simulink model "LKAS_Project"  (R2024b)
settings: Solver=ode45  StartTime=0.0  StopTime=T_final  RelTol=1e-3  EnableMultiTasking=on
undefined symbols (not defined in the file or in its folder): Calpha, Cf, Cr, driving, Izz, Kalpha, Ke, l, lf, lr, m, max_steer, mu, Tc, Vy0, X0, Y0, Yaw0, yaw_rate0
libraries: drivingscenarioandsensors x2
settings Model: Creator=user  LastModifiedBy=justi
settings SolverCC: ZeroCrossAlgorithm=Non-adaptive  AlgebraicLoopSolver=TrustRegion
settings DataIOCC: LimitDataPoints=on  SaveFormat=Array  SignalLoggingSaveFormat=ModelDataLogs  ReturnWorkspaceOutputs=off
settings OptimizationCC: ExpressionDepthLimit=2147483647  InitFltsAndDblsToZero=on  LifeSpan=inf
settings DebuggingCC: UnderspecifiedInitializationDetection=Classic  MergeDetectMultiDrivingBlocksExec=none  SolverPrmCheckMsg=warning  FcnCallInpInsideContextMsg=warning  UnconnectedInputMsg=warning  UnconnectedOutputMsg=warning  UnconnectedLineMsg=warning  StateNameClashWarn=warning  SFUnexpectedBacktrackingDiag=warning  SFNoUnconditionalDefaultTransitionDiag=warning  SFExecutionAtInitializationDiag=none  ArithmeticOperatorsInVariantConditions=warning
settings HardwareCC: ProdBitPerPointer=32  ProdBitPerSizeT=32  ProdBitPerPtrDiffT=32  ProdLargestAtomicFloat=None  ProdIntDivRoundTo=Undefined  ProdEndianess=Unspecified  ProdWordSize=32  ProdHWDeviceType=32-bit Generic
settings ModelReferenceCC: PropagateSignalLabelsOutOfModel=off
settings RTWCC: GPUComputeCapability=3.5
settings CodeAppCC: StateflowObjectComments=on
settings GRTTargetCC: TargetLangStandard=C89/C90 (ANSI)  CombineOutputUpdateFcns=off  GRTInterface=on
settings ConfigComp: CovMetricSettings=dw  CovSaveCumulativeToWorkspaceVar=on  CovSaveSingleToWorkspaceVar=on

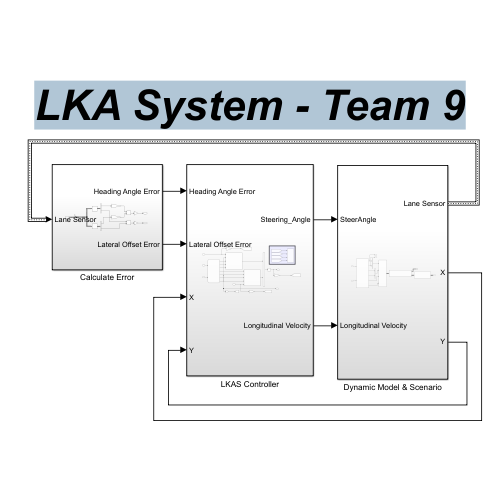
[thumbnail: Simulink's stored preview of the top-level diagram]
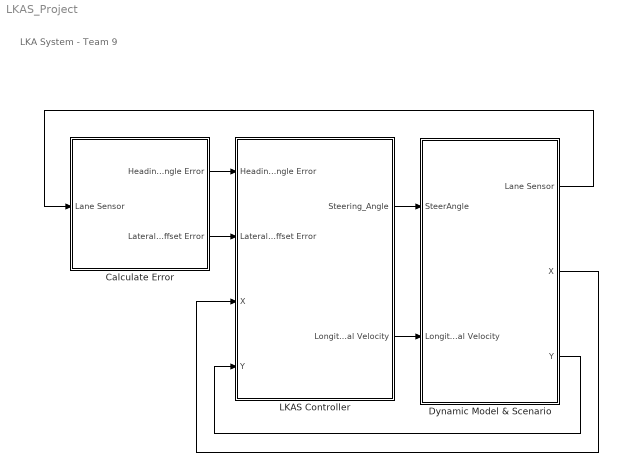
== system LKAS_Project ==
  note: LKA System - Team 9
  Calculate Error : Subsystem
  Dynamic Model & Scenario : Subsystem
  LKAS Controller : Subsystem
  wires:
  Dynamic Model & Scenario/1(Lane Sensor) -> Calculate Error/1(Lane Sensor)
  LKAS Controller/1(Steering_Angle) -> Dynamic Model & Scenario/1(SteerAngle)
  Dynamic Model & Scenario/2(X) -> LKAS Controller/3(X)
  Dynamic Model & Scenario/3(Y) -> LKAS Controller/4(Y)
  LKAS Controller/2(Longitudinal Velocity) -> Dynamic Model & Scenario/2(Longitudinal Velocity)
  Calculate Error/1(Heading Angle Error) -> LKAS Controller/1(Heading Angle Error)
  Calculate Error/2(Lateral Offset Error) -> LKAS Controller/2(Lateral Offset Error)

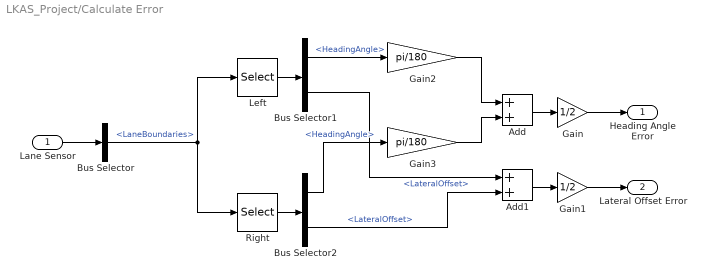
== system LKAS_Project/Calculate Error ==
  Lane Sensor : Inport
  Add : Sum
  Add1 : Sum
  Bus Selector : BusSelector  OutputSignals=LaneBoundaries
  Bus Selector1 : BusSelector  OutputSignals=HeadingAngle,LateralOffset
  Bus Selector2 : BusSelector  OutputSignals=HeadingAngle,LateralOffset
  Gain : Gain  Gain=1/2
  Gain1 : Gain  Gain=1/2
  Gain2 : Gain  Gain=pi/180
  Gain3 : Gain  Gain=pi/180
  Left : Selector  InputPortWidth=2  IndexOptions=Index vector (dialog)  Indices=[1]  OutputSizes=1
  Right : Selector  InputPortWidth=2  IndexOptions=Index vector (dialog)  Indices=[2]  OutputSizes=1
  Heading Angle Error : Outport
  Lateral Offset Error : Outport  Port=2
  wires:
  Add/1 -> Gain/1
  Bus Selector2/1 -> Gain3/1  "<HeadingAngle>"
  Bus Selector1/1 -> Gain2/1  "<HeadingAngle>"
  Add1/1 -> Gain1/1
  Bus Selector2/2 -> Add1/2  "<LateralOffset>"
  Bus Selector/1 -> Right/1, Left/1  "<LaneBoundaries>"
  Bus Selector1/2 -> Add1/1  "<LateralOffset>"
  Left/1 -> Bus Selector1/1
  Right/1 -> Bus Selector2/1
  Lane Sensor/1 -> Bus Selector/1
  Gain/1 -> Heading Angle Error/1
  Gain1/1 -> Lateral Offset Error/1
  Gain2/1 -> Add/1
  Gain3/1 -> Add/2

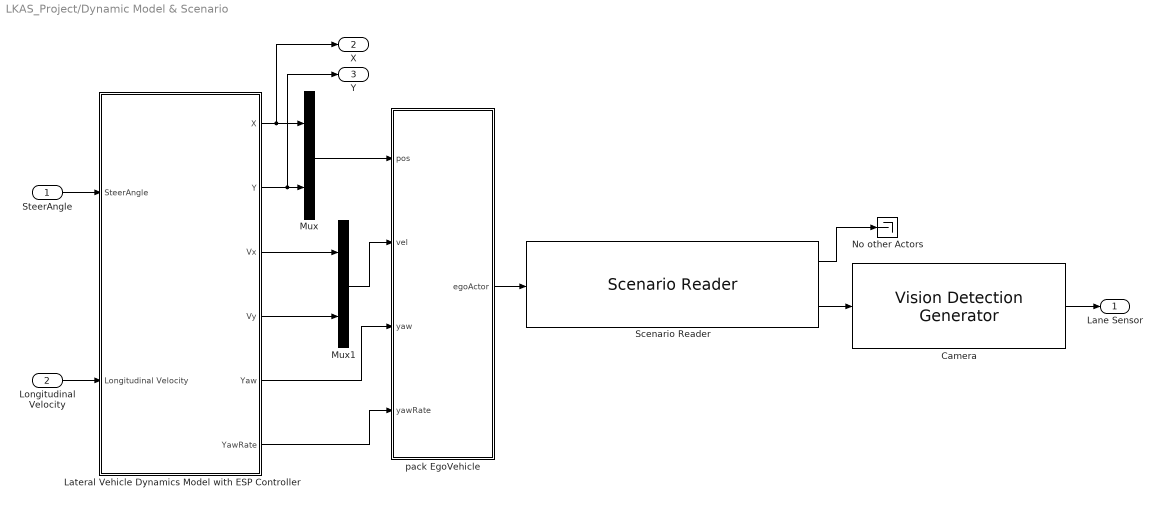
== system LKAS_Project/Dynamic Model & Scenario ==
  SteerAngle : Inport
  Longitudinal Velocity : Inport  Port=2
  Camera : drivingscenarioandsensors/Vision Detection Generator  SensorIndex=1  DetectorOutput=Lanes only  UpdateInterval=0.01  LaneUpdateInterval=0.1  SensorLocation=[1.9 0]  Height=1.1  Yaw=0  Pitch=1  Roll=0  BusNameSource=Auto  BusName=BusObjectDetections  BusName2Source=Property  BusName2=BusLaneDetections  MaxNumDetectionsSource=Property  MaxNumDetections=50  MaxNumLanesSource=Property  MaxNumLanes=2  DetectionCoordinates=Ego Cartesian  SimulateUsing=Interpreted execution  MaxRange=150  BoundingBoxAccuracy=5  ProcessNoiseIntensity=5  MaxSpeed=100  MaxAllowedOcclusion=0.5  MinObjectImageSize=[15 15]  DetectionProbability=0.9  FalsePositivesPerImage=0.1  MinLaneImageSize=[20 3]  LaneBoundaryAccuracy=3  HasNoise=on  InitialSeedSource=Repeatable  InitialSeed=0  UsedSeed=0  ActorProfilesSource=From Scenario Reader block  ActorProfilesParameters=driving.internal.ActorProfilesParameters  ActorProfilesExpression=[struct('ActorID',1,'ClassID',1,'Length',4.7,'Width',1.8,'Height',1.4,'OriginOffset',[-1.35 0 0],'MeshVertices',[3.7 0.9 0.857439446366782;3.7 -0.9 0.857439446366782;3.7 -0.9 0.314878892733564;3.7 0.9 0.314878892733564;3.7 0.9 0.857439446366782;2.525 0.9 0.993079584775086;2.525 -0.9 0.993079584775086;3.7 -0.9 0.857439446366782;1.82 0.72 1.4;0.41 0.72 1.4;0.41 -0.72 1.4;1.82 -0.72 1.4;-0.295 0.9 0.993079584775086;-1 0.9 0.857439446366782;-1 -0.9 0.857439446366782;-0.295 -0.9 0.993079584775086;3.7 0.9 0.857439446366782;3.7 0.9 0.314878892733564;2.525 0.9 0.314878892733564;2.525 0.9 0.993079584775086;2.525 0.9 0.993079584775086;2.525 0.9 0.314878892733564;-0.295 0.9 0.314878892733564;-0.295 0.9 0.993079584775086;-0.295 0.9 0.993079584775086;-0.295 0.9 0.314878892733564;-1 0.9 0.355570934256055;-1 0.9 0.857439446366782;2.525 0.9 0.993079584775086;-0.295 0.9 0.993079584775086;0.41 0.72 1.4;1.82 0.72 1.4;3.7 -0.9 0.857439446366782;3.7 -0.9 0.314878892733564;2.525 -0.9 0.314878892733564;2.525 -0.9 0.993079584775086;2.525 -0.9 0.993079584775086;2.525 -0.9 0.314878892733564;-0.295 -0.9 0.314878892733564;-0.295 -0.9 0.993079584775086;-0.295 -0.9 0.993079584775086;-0.295 -0.9 0.314878892733564;-1 -0.9 0.355570934256055;-1 -0.9 0.857439446366782;2.525 -0.9 0.993079584775086;-0.295 -0.9 0.993079584775086;0.41 -0.72 1.4;1.82 -0.72 1.4;-0.295 0.9 0.993079584775086;-0.295 -0.9 0.993079584775086;0.41 -0.72 1.4;0.41 0.72 1.4;2.525 -0.9 0.993079584775086;1.82 -0.72 1.4;1.82 0.72 1.4;2.525 0.9 0.993079584775086;-1 0.9 0.857439446366782;-1 0.9 0.355570934256055;-1 -0.9 0.355570934256055;-1 -0.9 0.857439446366782;3.7 0.9 0.314878892733564;3.7 -0.9 0.314878892733564;-0.295 -0.9 0.314878892733564;-0.295 0.9 0.314878892733564;-0.295 0.9 0.314878892733564;-1 0.9 0.355570934256055;-1 -0.9 0.355570934256055;-0.295 -0.9 0.314878892733564;0 -0.63 0;0 -0.87 0;0.191030206995054 -0.63 0.0601365173421445;0.191030206995054 -0.87 0.0601365173421445;0.309093367795925 -0.63 0.217575963708927;0.309093367795925 -0.87 0.217575963708927;0.309093367795925 -0.63 0.412181821758201;0.309093367795925 -0.87 0.412181821758201;0.191030206995054 -0.63 0.569621268124983;0.191030206995054 -0.87 0.569621268124983;0 -0.63 0.629757785467128;0 -0.87 0.629757785467128;-0.191030206995054 -0.63 0.569621268124983;-0.191030206995054 -0.87 0.569621268124983;-0.309093367795925 -0.63 0.412181821758201;-0.309093367795925 -0.87 0.412181821758201;-0.309093367795925 -0.63 0.217575963708927;-0.309093367795925 -0.87 0.217575963708927;-0.191030206995054 -0.63 0.0601365173421445;-0.191030206995054 -0.87 0.0601365173421445;0 -0.63 0;0 -0.87 0;0 -0.63 0;0.191030206995054 -0.63 0.0601365173421445;0.309093367795925 -0.63 0.217575963708927;0.309093367795925 -0.63 0.412181821758201;0.191030206995054 -0.63 0.569621268124983;0 -0.63 0.629757785467128;-0.191030206995054 -0.63 0.569621268124983;-0.309093367795925 -0.63 0.412181821758201;-0.309093367795925 -0.63 0.217575963708927;-0.191030206995054 -0.63 0.0601365173421445;0 -0.87 0;0.191030206995054 -0.87 0.0601365173421445;0.309093367795925 -0.87 0.217575963708927;0.309093367795925 -0.87 0.412181821758201;0.191030206995054 -0.87 0.569621268124983;0 -0.87 0.629757785467128;-0.191030206995054 -0.87 0.569621268124983;-0.309093367795925 -0.87 0.412181821758201;-0.309093367795925 -0.87 0.217575963708927;-0.191030206995054 -0.87 0.0601365173421445;0 0.87 0;0 0.63 0;0.191030206995054 0.87 0.0601365173421445;0.191030206995054 0.63 0.0601365173421445;0.309093367795925 0.87 0.217575963708927;0.309093367795925 0.63 0.217575963708927;0.309093367795925 0.87 0.412181821758201;0.309093367795925 0.63 0.412181821758201;0.191030206995054 0.87 0.569621268124983;0.191030206995054 0.63 0.569621268124983;0 0.87 0.629757785467128;0 0.63 0.629757785467128;-0.191030206995054 0.87 0.569621268124983;-0.191030206995054 0.63 0.569621268124983;-0.309093367795925 0.87 0.412181821758201;-0.309093367795925 0.63 0.412181821758201;-0.309093367795925 0.87 0.217575963708927;-0.309093367795925 0.63 0.217575963708927;-0.191030206995054 0.87 0.0601365173421445;-0.191030206995054 0.63 0.0601365173421445;0 ...(+3718 chars)],'MeshFaces',[1 2 3;3 4 1;5 6 7;7 8 5;9 10 11;11 12 9;13 14 15;15 16 13;17 18 19;19 20 17;21 22 23;23 24 21;25 26 27;27 28 25;29 30 31;31 32 29;33 34 35;35 36 33;37 38 39;39 40 37;41 42 43;43 44 41;45 46 47;47 48 45;49 50 51;51 52 49;53 54 55;55 56 53;57 58 59;59 60 57;61 62 63;63 64 61;65 66 67;67 68 65;69 71 72;72 70 69;71 73 74;74 72 71;73 75 76;76 74 73;75 77 78;78 76 75;77 79 80;80 78 77;79 81 82;82 80 79;81 83 84;84 82 81;83 85 86;86 84 83;85 87 88;88 86 85;87 89 90;90 88 87;91 92 93;91 93 94;91 94 95;91 95 96;91 96 97;91 97 98;91 98 99;91 99 100;101 102 103;101 103 104;101 104 105;101 105 106;101 106 107;101 107 108;101 108 109;101 109 110;111 113 114;114 112 111;113 115 116;116 114 113;115 117 118;118 116 115;117 119 120;120 118 117;119 121 122;122 120 119;121 123 124;124 122 121;123 125 126;126 124 123;125 127 128;128 126 125;127 129 130;130 128 127;129 131 132;132 130 129;133 134 135;133 135 136;133 136 137;133 137 138;133 138 139;133 139 140;133 140 141;133 141 142;143 144 145;143 145 146;143 146 147;143 147 148;143 148 149;143 149 150;143 150 151;143 151 152;153 155 156;156 154 153;155 157 158;158 156 155;157 159 160;160 158 157;159 161 162;162 160 159;161 163 164;164 162 161;163 165 166;166 164 163;165 167 168;168 166 165;167 169 170;170 168 167;169 171 172;172 170 169;171 173 174;174 172 171;175 176 177;175 177 178;175 178 179;175 179 180;175 180 181;175 181 182;175 182 183;175 183 184;185 186 187;185 187 188;185 188 189;185 189 190;185 190 191;185 191 192;185 192 193;185 193 194;195 197 198;198 196 195;197 199 200;200 198 197;199 201 202;202 200 199;201 203 204;204 202 201;203 205 206;206 204 203;205 207 208;208 206 205;207 209 210;210 208 207;209 211 212;212 210 209;211 213 214;214 212 211;213 215 216;216 214 213;217 218 219;217 219 220;217 220 221;217 221 222;217 222 223;217 223 224;217 224 225;217 225 226;227 228 229;227 229 230;227 230 231;227 231 232;227 232 233;227 233 234;227 234 235;227 235 236],'RCSPattern',[10 10;10 10],'RCSAzimuthAngles',[-180 180],'RCSElevationAngles',[-90 90])]  Intrinsics=driving.internal.cameraIntrinsics('FocalLength',[500 800],'PrincipalPoint',[320 240],'ImageSize',[480 640],'RadialDistortion',[0 0],'TangentialDistortion',[0 0],'Skew',0)
  Lateral Vehicle Dynamics Model with ESP Controller : Subsystem
  Mux : Mux  Inputs=2
  Mux1 : Mux  Inputs=2
  No other Actors : Terminator
  Scenario Reader : drivingscenarioandsensors/Scenario Reader  ScenarioSource=From file  ScenarioFileName="C:\\Users\\justi\\OneDrive\\바탕 화면\\국민대학교 자동차공학과  20203306 정혁주\\3학년 2학기\\자율주행 제어시스템 설계\\기말 프로젝트\\LKA_Project_9\\LKAS_9_Project_Scenario.mat"  ScenarioVariableName=scenario  OutputCoordinateSystem=Vehicle coordinates  EgoVehicleSource=Input port  EgoVehicleActorID=1  OrientVehiclesOnRoad=off  OutputEgoVehiclePose=off  OutputEgoVehicleState=off  SampleTime=0.1  LaneBoundaryOutput=Ego vehicle lane boundaries  LaneBoundaryDistance=0:1:30  LaneBoundaryLocation=Center of lane markings  BusNameSource=Auto  BusName=BusActors  BusNumActorsSource=Scenario  BusNumActors=100  BusName2Source=Auto  BusName2=BusLaneBoundaries  BusNumLaneBoundariesSource=Scenario  BusNumLaneBoundaries=10  BusName3Source=Auto  BusName3=BusEgoActor  BusName4Source=Auto  BusName4=BusEgoState  ShowCoordinateLabels=on  SimulateUsing=Interpreted execution
  pack EgoVehicle : MATLAB Function  TreatAsAtomicUnit=on
  Lane Sensor : Outport
  X : Outport  Port=2
  Y : Outport  Port=3
  wires:
  Lateral Vehicle Dynamics Model with ESP Controller/2(Y) -> Y/1, Mux/2
  Lateral Vehicle Dynamics Model with ESP Controller/4(Vy) -> Mux1/2
  Mux/1 -> pack EgoVehicle/1(pos)
  Lateral Vehicle Dynamics Model with ESP Controller/3(Vx) -> Mux1/1
  Mux1/1 -> pack EgoVehicle/2(vel)
  Lateral Vehicle Dynamics Model with ESP Controller/6(YawRate) -> pack EgoVehicle/4(yawRate)
  Lateral Vehicle Dynamics Model with ESP Controller/5(Yaw) -> pack EgoVehicle/3(yaw)
  Lateral Vehicle Dynamics Model with ESP Controller/1(X) -> X/1, Mux/1
  Scenario Reader/1 -> No other Actors/1
  pack EgoVehicle/1(egoActor) -> Scenario Reader/1
  Scenario Reader/2 -> Camera/1
  Camera/1 -> Lane Sensor/1
  SteerAngle/1 -> Lateral Vehicle Dynamics Model with ESP Controller/1(SteerAngle)
  Longitudinal Velocity/1 -> Lateral Vehicle Dynamics Model with ESP Controller/2(Longitudinal Velocity)

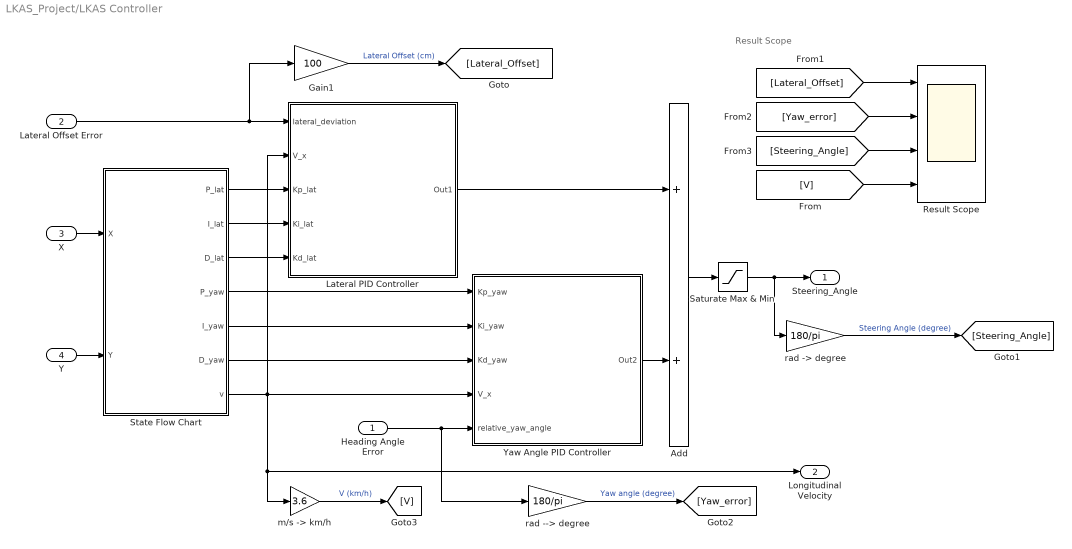
== system LKAS_Project/LKAS Controller ==
  note: Result Scope
  Heading Angle Error : Inport
  Lateral Offset Error : Inport  Port=2
  X : Inport  Port=3
  Y : Inport  Port=4
  Add : Sum
  Gain1 : Gain  Gain=100
  Lateral PID Controller : Subsystem
  Result Scope : Scope  NumInputPorts=4
  Saturate Max & Min : Saturate  UpperLimit=max_steer  LowerLimit=-max_steer  LinearizeAsGain=off
  State Flow Chart : Stateflow chart  TreatAsAtomicUnit=on
  Yaw Angle PID Controller : Subsystem
  "m/s -> km/h" : Gain  Gain=3.6
  rad --> degree : Gain  Gain=180/pi
  "rad -> degree" : Gain  Gain=180/pi
  Steering_Angle : Outport
  Longitudinal Velocity : Outport  Port=2
  wires:
  Yaw Angle PID Controller/1(Out2) -> Add/2
  Lateral PID Controller/1(Out1) -> Add/1
  Add/1 -> Saturate Max & Min/1
  Heading Angle Error/1 -> rad --> degree/1, Yaw Angle PID Controller/5(relative_yaw_angle)
  Lateral Offset Error/1 -> Gain1/1, Lateral PID Controller/1(lateral_deviation)
  Saturate Max & Min/1 -> Steering_Angle/1, "rad -> degree"/1
  X/1 -> State Flow Chart/1(X)
  Y/1 -> State Flow Chart/2(Y)
  State Flow Chart/7(v) -> "m/s -> km/h"/1, Longitudinal Velocity/1, Lateral PID Controller/2(V_x), Yaw Angle PID Controller/4(V_x)
  rad --> degree/1 -> [Yaw_error]  "Yaw angle (degree)"
  Gain1/1 -> [Lateral_Offset]  "Lateral Offset (cm)"
  "rad -> degree"/1 -> [Steering_Angle]  "Steering Angle (degree)"
  State Flow Chart/1(P_lat) -> Lateral PID Controller/3(Kp_lat)
  State Flow Chart/2(I_lat) -> Lateral PID Controller/4(Ki_lat)
  State Flow Chart/3(D_lat) -> Lateral PID Controller/5(Kd_lat)
  State Flow Chart/4(P_yaw) -> Yaw Angle PID Controller/1(Kp_yaw)
  State Flow Chart/5(I_yaw) -> Yaw Angle PID Controller/2(Ki_yaw)
  State Flow Chart/6(D_yaw) -> Yaw Angle PID Controller/3(Kd_yaw)
  [V] -> Result Scope/4
  [Lateral_Offset] -> Result Scope/1
  [Yaw_error] -> Result Scope/2
  [Steering_Angle] -> Result Scope/3
  "m/s -> km/h"/1 -> [V]  "V (km/h)"

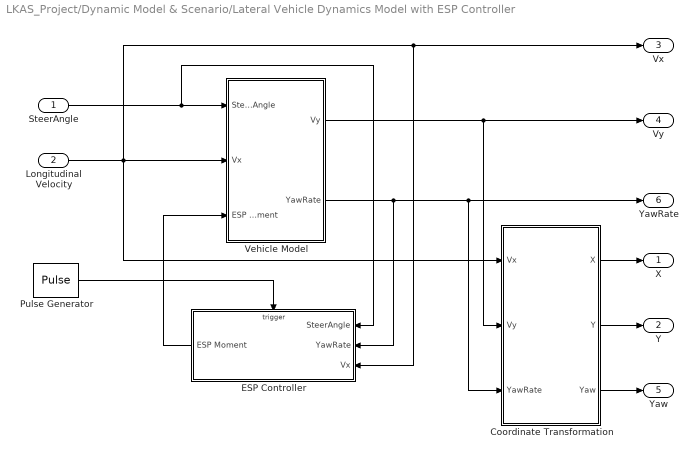
== system LKAS_Project/Dynamic Model & Scenario/Lateral Vehicle Dynamics Model with ESP Controller ==
  SteerAngle : Inport
  Longitudinal Velocity : Inport  Port=2
  Coordinate Transformation : Subsystem
  ESP Controller : Subsystem
  Pulse Generator : DiscretePulseGenerator  PulseType=Time based  Period=Tc  PulseWidth=50
  Vehicle Model : Subsystem
  X : Outport
  Y : Outport  Port=2
  Vx : Outport  Port=3
  Vy : Outport  Port=4
  Yaw : Outport  Port=5
  YawRate : Outport  Port=6
  wires:
  Vehicle Model/1(Vy) -> Vy/1, Coordinate Transformation/2(Vy)
  Vehicle Model/2(YawRate) -> YawRate/1, Coordinate Transformation/3(YawRate), ESP Controller/2(YawRate)
  Longitudinal Velocity/1 -> Vehicle Model/2(Vx), Vx/1, ESP Controller/3(Vx), Coordinate Transformation/1(Vx)
  SteerAngle/1 -> Vehicle Model/1(Steering_Angle), ESP Controller/1(SteerAngle)
  Pulse Generator/1 -> ESP Controller/Trigger
  Coordinate Transformation/1(X) -> X/1
  ESP Controller/1(ESP Moment) -> Vehicle Model/3(ESP Moment)
  Coordinate Transformation/2(Y) -> Y/1
  Coordinate Transformation/3(Yaw) -> Yaw/1

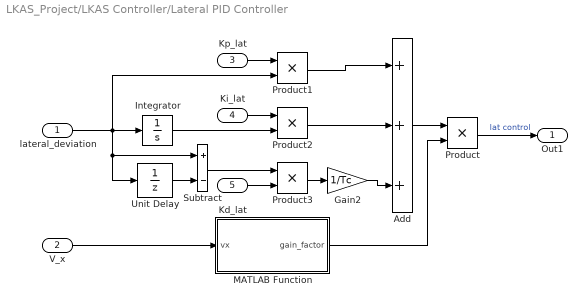
== system LKAS_Project/LKAS Controller/Lateral PID Controller ==
  lateral_deviation : Inport
  V_x : Inport  Port=2
  Kp_lat : Inport  Port=3
  Ki_lat : Inport  Port=4
  Kd_lat : Inport  Port=5
  Add : Sum  Inputs=+++
  Gain2 : Gain  Gain=1/Tc
  Integrator : Integrator
  MATLAB Function : MATLAB Function  TreatAsAtomicUnit=on
  Product{,1..3} (4 alike) : Product
  Subtract : Sum  Inputs=+-
  Unit Delay : UnitDelay  SampleTime=Tc  HasFrameUpgradeWarning=on
  Out1 : Outport
  wires:
  Integrator/1 -> Product2/2
  lateral_deviation/1 -> Product1/2, Subtract/1, Unit Delay/1, Integrator/1
  Subtract/1 -> Product3/1
  Product1/1 -> Add/1
  Gain2/1 -> Add/3
  Unit Delay/1 -> Subtract/2
  Add/1 -> Product/1
  V_x/1 -> MATLAB Function/1(vx)
  MATLAB Function/1(gain_factor) -> Product/2
  Product/1 -> Out1/1  "lat control"
  Product2/1 -> Add/2
  Kp_lat/1 -> Product1/1
  Ki_lat/1 -> Product2/1
  Product3/1 -> Gain2/1
  Kd_lat/1 -> Product3/2

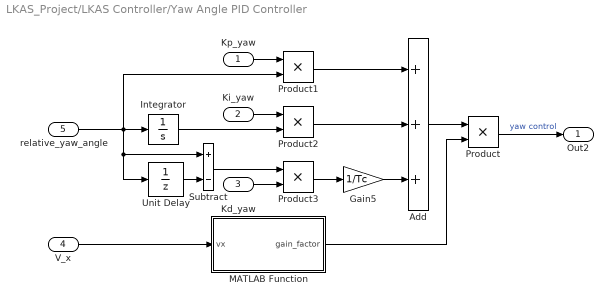
== system LKAS_Project/LKAS Controller/Yaw Angle PID Controller ==
  Kp_yaw : Inport
  Ki_yaw : Inport  Port=2
  Kd_yaw : Inport  Port=3
  V_x : Inport  Port=4
  relative_yaw_angle : Inport  Port=5
  Add : Sum  Inputs=+++
  Gain5 : Gain  Gain=1/Tc
  Integrator : Integrator
  MATLAB Function : MATLAB Function  TreatAsAtomicUnit=on
  Product{,1..3} (4 alike) : Product
  Subtract : Sum  Inputs=+-
  Unit Delay : UnitDelay  SampleTime=Tc  HasFrameUpgradeWarning=on
  Out2 : Outport
  wires:
  Product/1 -> Out2/1  "yaw control"
  Subtract/1 -> Product3/1
  Add/1 -> Product/1
  Unit Delay/1 -> Subtract/2
  Integrator/1 -> Product2/2
  Product2/1 -> Add/2
  V_x/1 -> MATLAB Function/1(vx)
  MATLAB Function/1(gain_factor) -> Product/2
  relative_yaw_angle/1 -> Product1/2, Integrator/1, Subtract/1, Unit Delay/1
  Gain5/1 -> Add/3
  Product1/1 -> Add/1
  Kp_yaw/1 -> Product1/1
  Ki_yaw/1 -> Product2/1
  Product3/1 -> Gain5/1
  Kd_yaw/1 -> Product3/2

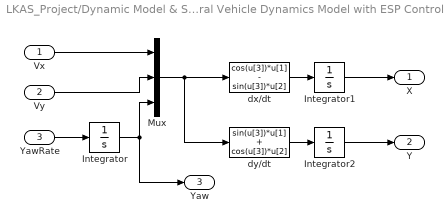
== system LKAS_Project/Dynamic Model & Scenario/Lateral Vehicle Dynamics Model with ESP Controller/Coordinate Transformation ==
  Vx : Inport
  Vy : Inport  Port=2
  YawRate : Inport  Port=3
  Integrator : Integrator  InitialCondition=Yaw0
  Integrator1 : Integrator  InitialCondition=X0
  Integrator2 : Integrator  InitialCondition=Y0
  Mux : Mux  Inputs=3
  dx/dt : Fcn  Expr=cos(u[3])*u[1] - sin(u[3])*u[2]
  dy/dt : Fcn  Expr=sin(u[3])*u[1] + cos(u[3])*u[2]
  X : Outport
  Y : Outport  Port=2
  Yaw : Outport  Port=3
  wires:
  YawRate/1 -> Integrator/1
  Vx/1 -> Mux/1
  Vy/1 -> Mux/2
  Integrator/1 -> Mux/3, Yaw/1
  Mux/1 -> dx/dt/1, dy/dt/1
  dx/dt/1 -> Integrator1/1
  Integrator1/1 -> X/1
  dy/dt/1 -> Integrator2/1
  Integrator2/1 -> Y/1

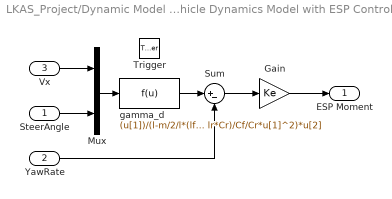
== system LKAS_Project/Dynamic Model & Scenario/Lateral Vehicle Dynamics Model with ESP Controller/ESP Controller ==
  SteerAngle : Inport
  YawRate : Inport  Port=2
  Vx : Inport  Port=3
  Trigger : TriggerPort  VariantControl=(inherit)
  Gain : Gain  Gain=Ke
  Mux : Mux  Inputs=2
  Sum : Sum  Inputs=|+-
  gamma_d : Fcn  Expr=(u[1])/(l-m/2/l*(lf*Cf - lr*Cr)/Cf/Cr*u[1]^2)*u[2]
  ESP Moment : Outport
  wires:
  Vx/1 -> Mux/1
  SteerAngle/1 -> Mux/2
  Mux/1 -> gamma_d/1
  gamma_d/1 -> Sum/1
  YawRate/1 -> Sum/2
  Sum/1 -> Gain/1
  Gain/1 -> ESP Moment/1

== system LKAS_Project/Dynamic Model & Scenario/Lateral Vehicle Dynamics Model with ESP Controller/Vehicle Model ==
  Steering_Angle : Inport
  Vx : Inport  Port=2
  ESP Moment : Inport  Port=3
  Bicycle Model : Subsystem
  Lateral Tire Model : Subsystem
  Vy : Outport
  YawRate : Outport  Port=2
  wires:
  Steering_Angle/1 -> Lateral Tire Model/2(SteeringAngle)
  Lateral Tire Model/1(Front Lateral Tire Force) -> Bicycle Model/1(Front lateral tire force)
  Lateral Tire Model/2(Rear Lateral Tire Force) -> Bicycle Model/2(Rear lateral tire force)
  Bicycle Model/1(YawRate) -> YawRate/1, Lateral Tire Model/1(YawRate)
  Bicycle Model/2(Vy) -> Vy/1, Lateral Tire Model/4(Vy)
  Vx/1 -> Lateral Tire Model/3(Vx), Bicycle Model/3(Vx)
  ESP Moment/1 -> Bicycle Model/4(ESP Moment)

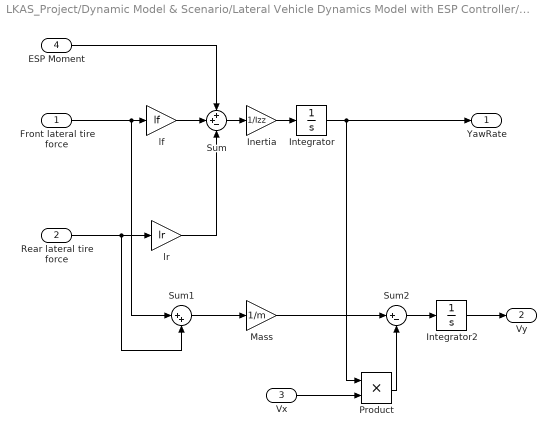
== system LKAS_Project/Dynamic Model & Scenario/Lateral Vehicle Dynamics Model with ESP Controller/Vehicle Model/Bicycle Model ==
  Front lateral tire force : Inport
  Rear lateral tire force : Inport  Port=2
  Vx : Inport  Port=3
  ESP Moment : Inport  Port=4
  Inertia : Gain  Gain=1/Izz
  Integrator : Integrator  InitialCondition=yaw_rate0
  Integrator2 : Integrator  InitialCondition=Vy0
  Mass : Gain  Gain=1/m
  Product : Product  RndMeth=Zero
  Sum : Sum  Inputs=++-
  Sum1 : Sum  Inputs=|++
  Sum2 : Sum  Inputs=|+-
  lf : Gain  Gain=lf
  lr : Gain  Gain=lr
  YawRate : Outport
  Vy : Outport  Port=2
  wires:
  Front lateral tire force/1 -> lf/1, Sum1/1
  Rear lateral tire force/1 -> lr/1, Sum1/2
  Sum/1 -> Inertia/1
  Inertia/1 -> Integrator/1
  Integrator/1 -> YawRate/1, Product/1
  Sum1/1 -> Mass/1
  Mass/1 -> Sum2/1
  Vx/1 -> Product/2
  Product/1 -> Sum2/2
  Sum2/1 -> Integrator2/1
  Integrator2/1 -> Vy/1
  ESP Moment/1 -> Sum/1
  lf/1 -> Sum/2
  lr/1 -> Sum/3

== system LKAS_Project/Dynamic Model & Scenario/Lateral Vehicle Dynamics Model with ESP Controller/Vehicle Model/Lateral Tire Model ==
  YawRate : Inport
  SteeringAngle : Inport  Port=2
  Vx : Inport  Port=3
  Vy : Inport  Port=4
  Front Tire Model : Subsystem
  Rear Tire Model : Subsystem
  Front Lateral Tire Force : Outport
  Rear Lateral Tire Force : Outport  Port=2
  wires:
  Vx/1 -> Rear Tire Model/2(Vx), Front Tire Model/2(Vx)
  Vy/1 -> Rear Tire Model/3(Vy), Front Tire Model/3(Vy)
  YawRate/1 -> Front Tire Model/1(YawRate), Rear Tire Model/1(YawRate)
  Front Tire Model/1(Front Lateral Tire Force) -> Front Lateral Tire Force/1
  SteeringAngle/1 -> Front Tire Model/4(Steering Angle)
  Rear Tire Model/1(Rear Lateral Tire Force) -> Rear Lateral Tire Force/1

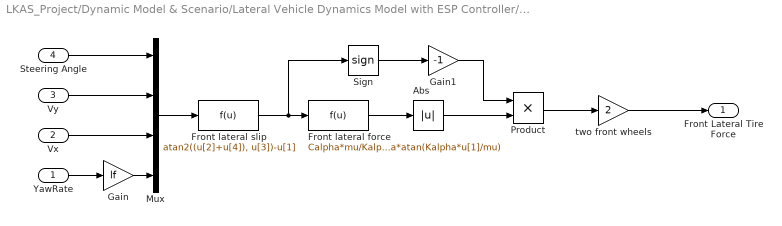
== system LKAS_Project/Dynamic Model & Scenario/Lateral Vehicle Dynamics Model with ESP Controller/Vehicle Model/Lateral Tire Model/Front Tire Model ==
  YawRate : Inport
  Vx : Inport  Port=2
  Vy : Inport  Port=3
  Steering Angle : Inport  Port=4
  Abs : Abs  SaturateOnIntegerOverflow=off
  Front lateral force : Fcn  Expr=Calpha*mu/Kalpha*atan(Kalpha*u[1]/mu)
  Front lateral slip : Fcn  Expr=atan2((u[2]+u[4]), u[3])-u[1]
  Gain : Gain  Gain=lf
  Gain1 : Gain  Gain=-1
  Mux : Mux
  Product : Product  RndMeth=Zero
  Sign : Signum
  two front wheels : Gain  Gain=2
  Front Lateral Tire Force : Outport
  wires:
  Steering Angle/1 -> Mux/1
  Vy/1 -> Mux/2
  Vx/1 -> Mux/3
  YawRate/1 -> Gain/1
  Mux/1 -> Front lateral slip/1
  Gain/1 -> Mux/4
  Front lateral slip/1 -> Front lateral force/1, Sign/1
  Front lateral force/1 -> Abs/1
  Sign/1 -> Gain1/1
  Gain1/1 -> Product/1
  Abs/1 -> Product/2
  Product/1 -> two front wheels/1
  two front wheels/1 -> Front Lateral Tire Force/1

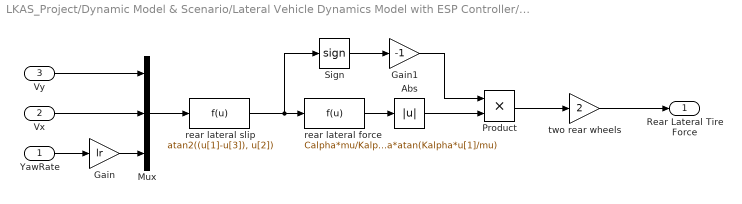
== system LKAS_Project/Dynamic Model & Scenario/Lateral Vehicle Dynamics Model with ESP Controller/Vehicle Model/Lateral Tire Model/Rear Tire Model ==
  YawRate : Inport
  Vx : Inport  Port=2
  Vy : Inport  Port=3
  Abs : Abs  SaturateOnIntegerOverflow=off
  Gain : Gain  Gain=lr
  Gain1 : Gain  Gain=-1
  Mux : Mux  Inputs=3
  Product : Product  RndMeth=Zero
  Sign : Signum
  rear lateral force : Fcn  Expr=Calpha*mu/Kalpha*atan(Kalpha*u[1]/mu)
  rear lateral slip : Fcn  Expr=atan2((u[1]-u[3]), u[2])
  two rear wheels : Gain  Gain=2
  Rear Lateral Tire Force : Outport
  wires:
  rear lateral slip/1 -> rear lateral force/1, Sign/1
  Gain/1 -> Mux/3
  Mux/1 -> rear lateral slip/1
  YawRate/1 -> Gain/1
  Vy/1 -> Mux/1
  Vx/1 -> Mux/2
  Sign/1 -> Gain1/1
  rear lateral force/1 -> Abs/1
  Gain1/1 -> Product/1
  Abs/1 -> Product/2
  Product/1 -> two rear wheels/1
  two rear wheels/1 -> Rear Lateral Tire Force/1

== matlab function LKAS_Project/LKAS Controller/Yaw Angle PID Controller/MATLAB Function ==
  data: vx input; gain_factor output
function gain_factor = calculateGain(vx)
% Gain adjustment function according to vehicle speed / gain_factor : between 0 and 1

    % parameters
    Cf = 38925;
    m = 2045;
    l = 3.2;
    
    % If the speed is 0, the gain factor is set to 1
    if vx <= 0
        gain_factor = 1.0;
        return;
    end

    velocity_scale = sqrt((Cf * l^2) / (m * vx^2));
    
    % Minimum limit
    gain_factor = min(1.0, velocity_scale);
end

== matlab function LKAS_Project/Dynamic Model & Scenario/pack EgoVehicle ==
  data: pos input; egoActor output Bus: BusActors1Actors size=1; vel input; yaw input; yawRate input
function egoActor = packEgo(pos, vel, yaw, yawRate)

egoActor = struct(...
    'ActorID', 1,...
    'Position', [pos(1) pos(2) 0], ...
    'Velocity', [vel(1) vel(2) 0], ...
    'Roll', 0, ...
    'Pitch', 0, ...
    'Yaw', rad2deg(yaw), ...
    'AngularVelocity', [0 0 rad2deg(yawRate)]);

== stateflow chart LKAS_Project/LKAS Controller/State Flow Chart ==
  state Speed_25
    entry:
    v = 25/3.6
    P_lat = 0.8;
    I_lat = 0.005;
    D_lat = 0.25;
    P_yaw = 1.2;
    I_yaw = 0.01;
    D_yaw = 0.3;
  state Speed_15
    entry:
    v = 15/3.6;
    P_lat = 0.7;
    I_lat = 0.3;
    D_lat = 0.2;
    P_yaw = 1.15;
    I_yaw = 0.3;
    D_yaw = 0.25;
  state Speed_30
    entry:
    v = 30/3.6;
    P_lat = 0.4;
    I_lat = 0.05;
    D_lat = 0.2;
    P_yaw = 1.0;
    I_yaw = 0.25;
    D_yaw = 0.35;
  state Speed_20
    entry:
    v = 20/3.6;
    P_lat = 1.5;
    I_lat = 0.05;
    D_lat = 0.2;
    P_yaw = 1.0;
    I_yaw = 0.05;
    D_yaw = 0.3;
  Speed_30 -> Speed_25 [order 1] : [check_position(X, Y, 50, 0, 3.0)]
  Speed_25 -> Speed_20 : [[check_position(X, Y, 250, 100, 3.0)] || ...
      |  [check_position(X, Y, 350, 250, 3.0)] || ...
      | [check_position(X, Y, 0, 200, 3.0)]]
  Speed_20 -> Speed_25 [order 3] : [[check_position(X, Y, 350, 200, 3.0)] || ...
      | [check_position(X, Y, 150, 200, 3.0)]]
  (default) -> Speed_30
  Speed_15 -> Speed_20 : [check_position(X, Y, 250, 300, 3.0)]
  Speed_20 -> Speed_30 [order 1] : [check_position(X, Y, 0, 0, 3.0)]
  Speed_20 -> Speed_15 [order 2] : [check_position(X, Y, 350, 300, 3.0)]
  Speed_30 -> Speed_20 [order 2] : [check_position(X, Y, 350, 300, 3.0)]
  data: x function_input; y function_input; target_x function_input; target_y function_input; tolerance function_input; is_within_range function_output; P_lat output; I_lat output; D_lat output; X input; Y input; P_yaw output; I_yaw output; D_yaw output; v output
  function is_within_range = check_position(x, y, target_x, target_y, tolerance):
    | function is_within_range = check_position(x, y, target_x, target_y, tolerance)
    |     % x, y: 현재 위치 / target_x, target_y: 목표 위치 / tolerance: 허용 오차
    | 
    |     if abs(x - target_x) <= tolerance && abs(y - target_y) <= tolerance
    |         is_within_range = true;
    |     else
    |         is_within_range = false;
    |     end
    | end

== matlab function LKAS_Project/LKAS Controller/Lateral PID Controller/MATLAB Function ==
  data: vx input; gain_factor output
function gain_factor = calculateGain(vx)
% Gain adjustment function according to vehicle speed / gain_factor : between 0 and 1

    % parameters
    Cf = 38925;
    m = 2045;
    l = 3.2;
    
    % If the speed is 0, the gain factor is set to 1
    if vx <= 0
        gain_factor = 1.0;
        return;
    end

    velocity_scale = sqrt((Cf * l^2) / (m * vx^2));
    
    % Minimum limit
    gain_factor = min(1.0, velocity_scale);
end
